simulink model "termproject"  (R2022b)
settings: Solver=VariableStepAuto  StartTime=0.0  StopTime=300  RelTol=1e-3
libraries: vrlib x4, simulink x1
settings Model: NumberOfSteps=10  PacingRate=0.280000  Creator=채준희  LastModifiedBy=채준희

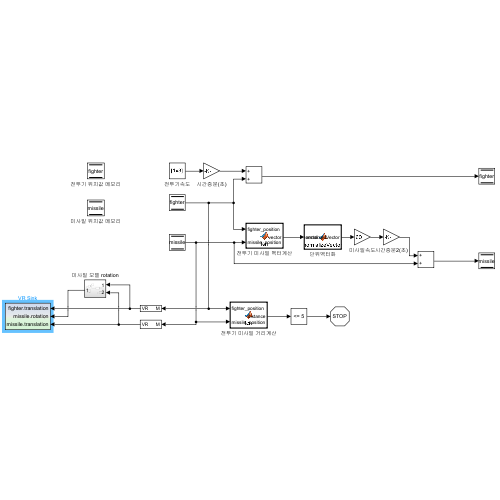
[thumbnail: Simulink's stored preview of the top-level diagram]
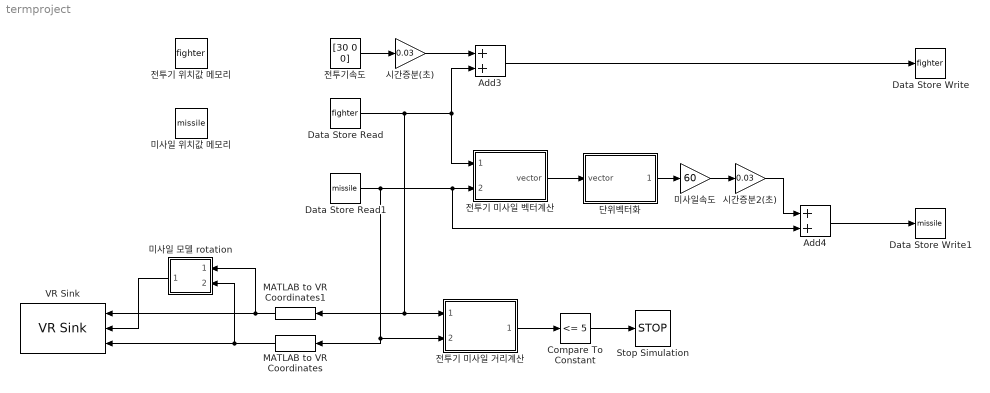
== system termproject ==
  Add3 : Sum
  Add4 : Sum
  Compare To Constant : simulink/Logic and Bit Operations/Compare To Constant  relop=<=  const=5  OutDataTypeStr=boolean
  Data Store Read : DataStoreRead  DataStoreName=fighter  IndexOptions=Index vector (dialog)  Indices=1  OutputSizes=1
  Data Store Read1 : DataStoreRead  DataStoreName=missile  IndexOptions=Index vector (dialog)  Indices=1  OutputSizes=1
  Data Store Write : DataStoreWrite  DataStoreName=fighter  IndexOptions=Index vector (dialog)  Indices=1  OutputSizes=1
  Data Store Write1 : DataStoreWrite  DataStoreName=missile  IndexOptions=Index vector (dialog)  Indices=1  OutputSizes=1
  MATLAB to VR Coordinates : vrlib/Utilities/MATLAB to VR Coordinates
  MATLAB to VR Coordinates1 : vrlib/Utilities/MATLAB to VR Coordinates
  Stop Simulation : Stop
  VR Sink : vrlib/VR Sink  InstantiateOnLoad=on  SampleTime=0.1  ViewEnable=on  RemoteChange=off  RemoteView=off  FieldsWritten=fighter.translation.3.1.1.double#missile.rotation.4.1.1.double#missile.translation.3.1.1.double  WorldFileName=termproject_3d.x3d  AutoView=off  VideoDimensions=[]  AllowVariableSize=off
  단위벡터화 : MATLAB Function  TreatAsAtomicUnit=on
  미사일 모델 rotation : Subsystem
  미사일 위치값 메모리 : DataStoreMemory  DataStoreName=missile  WriteAfterWriteMsg=warning  InitialValue=[500 0 0 ]  VectorParams1D=off  ShowAdditionalParam=off
  미사일속도 : Gain  Gain=60
  시간증분(초) : Gain  Gain=0.03
  시간증분2(초) : Gain  Gain=0.03
  전투기 미사일 거리계산 : MATLAB Function  TreatAsAtomicUnit=on
  전투기 미사일 벡터계산 : MATLAB Function  TreatAsAtomicUnit=on
  전투기 위치값 메모리 : DataStoreMemory  DataStoreName=fighter  WriteAfterWriteMsg=warning  InitialValue=[0 0 100]  VectorParams1D=off  ShowAdditionalParam=off
  전투기속도 : Constant  Value=[30 0 0]  VectorParams1D=off
  wires:
  Data Store Read/1 -> 전투기 미사일 거리계산/1(fighter_position), MATLAB to VR Coordinates1/1, Add3/2, 전투기 미사일 벡터계산/1(fighter_position)
  전투기속도/1 -> 시간증분(초)/1
  Add3/1 -> Data Store Write/1
  Data Store Read1/1 -> MATLAB to VR Coordinates/1, 전투기 미사일 거리계산/2(missile_position), 전투기 미사일 벡터계산/2(missile_position), Add4/2
  전투기 미사일 벡터계산/1(vector) -> 단위벡터화/1(vector)
  단위벡터화/1(normalizedVector) -> 미사일속도/1
  Add4/1 -> Data Store Write1/1
  미사일속도/1 -> 시간증분2(초)/1
  전투기 미사일 거리계산/1(distance) -> Compare To Constant/1
  Compare To Constant/1 -> Stop Simulation/1
  시간증분(초)/1 -> Add3/1
  시간증분2(초)/1 -> Add4/1
  MATLAB to VR Coordinates/1 -> 미사일 모델 rotation/2(In2), VR Sink/3
  MATLAB to VR Coordinates1/1 -> VR Sink/1, 미사일 모델 rotation/1(In1)
  미사일 모델 rotation/1(Out1) -> VR Sink/2

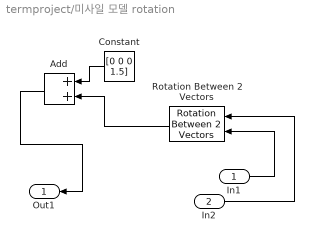
== system termproject/미사일 모델 rotation ==
  In1 : Inport
  In2 : Inport  Port=2
  Add : Sum
  Constant : Constant  Value=[0 0 0 1.5]
  Rotation Between 2 Vectors : vrlib/Utilities/Rotation Between 2 Vectors
  Out1 : Outport
  wires:
  Constant/1 -> Add/1
  Rotation Between 2 Vectors/1 -> Add/2
  In2/1 -> Rotation Between 2 Vectors/1
  In1/1 -> Rotation Between 2 Vectors/2
  Add/1 -> Out1/1

== matlab function termproject/전투기 미사일 벡터계산 ==
  data: fighter_position input; vector output; missile_position input
function vector = fcn(fighter_position,missile_position)
vector=[fighter_position(1)-missile_position(1),fighter_position(2)-missile_position(2),fighter_position(3)-missile_position(3)];

end

== matlab function termproject/단위벡터화 ==
  data: vector input; normalizedVector output
function normalizedVector  = normalizeVector(vector)
    magnitude = norm(vector);
    if magnitude ~= 0
        normalizedVector = vector / magnitude;
    else
        normalizedVector = vector;
    end
end

== matlab function termproject/전투기 미사일 거리계산 ==
  data: fighter_position input; distance output; missile_position input
function distance = fcn(fighter_position,missile_position)
distance=sqrt(((fighter_position(1)-missile_position(1))^2)+((fighter_position(2)-missile_position(2))^2)+((fighter_position(3)-missile_position(3))^2));

end
